simulink model "Ejercicios"  (R2023b)
settings: Solver=VariableStepAuto  StartTime=0.0  StopTime=5  MaxStep=1e-5  RelTol=1e-3
libraries: spsRMSLib x16, spsSeriesRLCBranchLib x12, spsVoltageMeasurementLib x9, spsCurrentMeasurementLib x6, spsPowerLib x6, spsACVoltageSourceLib x3, spsControlledVoltageSourceLib x2, spsDCVoltageSourceLib x1, spsDetailedThyristorLib x1, spsMutualInductanceLib x1, spsTHDLib x1, sps_lib x1
settings Model: Creator=Usuario_UMA  LastModifiedBy=Usuario_UMA

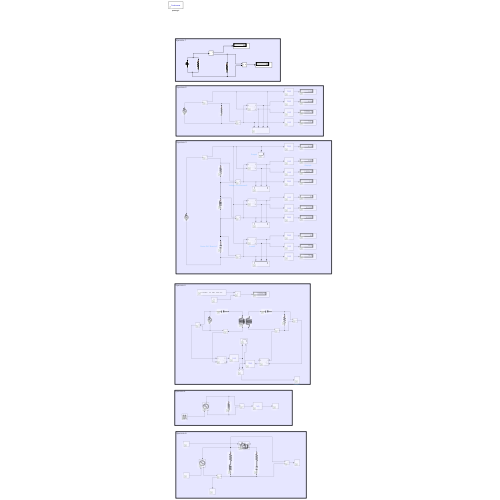
[thumbnail: Simulink's stored preview of the top-level diagram]
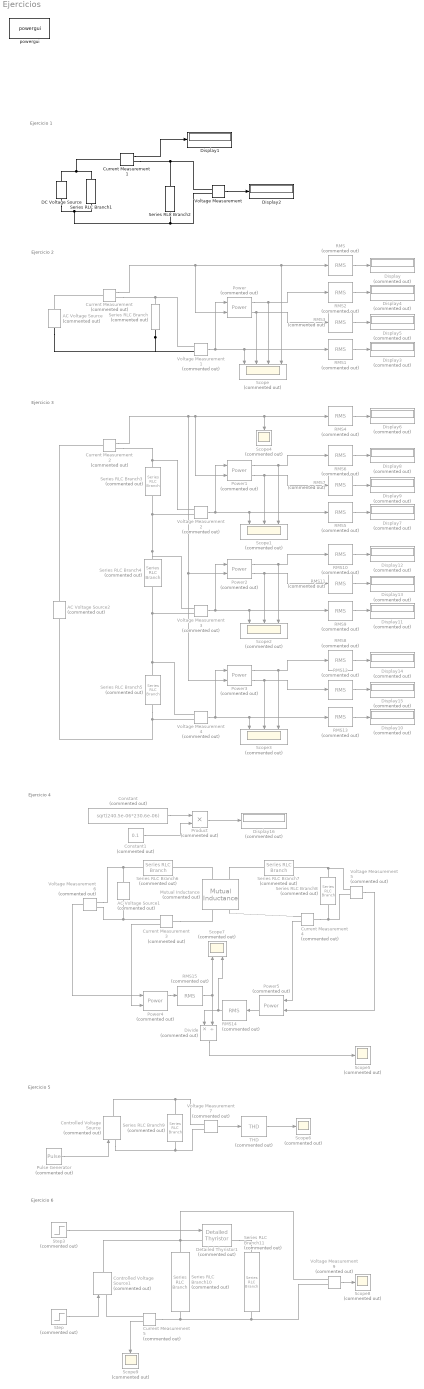
== system Ejercicios ==
  note: Ejercicio 6
  note: Ejercicio 5
  note: Ejercicio 4
  note: Ejercicio 2
  note: Ejercicio 1
  note: Ejercicio 3
  AC Voltage Source : spsACVoltageSourceLib/AC Voltage Source  Commented=on  Amplitude=10  Phase=0  Frequency=50  SampleTime=0  Measurements=None  BusType=swing  Pref=10e3  Qref=0  Qmin=-inf  Qmax=+inf
  AC Voltage Source1 : spsACVoltageSourceLib/AC Voltage Source  Commented=on  Amplitude=300  Phase=0  Frequency=85000  SampleTime=0  Measurements=None  BusType=swing  Pref=10e3  Qref=0  Qmin=-inf  Qmax=+inf
  AC Voltage Source2 : spsACVoltageSourceLib/AC Voltage Source  Commented=on  Amplitude=100  Phase=0  Frequency=50  SampleTime=0  Measurements=None  BusType=swing  Pref=10e3  Qref=0  Qmin=-inf  Qmax=+inf
  Constant : Constant  Commented=on  Value=sqrt(240.5e-06*230.6e-06)
  Constant1 : Constant  Commented=on  Value=0.1
  Controlled Voltage Source : spsControlledVoltageSourceLib/Controlled Voltage Source  Commented=on  Initialize=on  Source_Type=AC  Amplitude=0  Phase=0  Frequency=0  Measurements=None
  Controlled Voltage Source1 : spsControlledVoltageSourceLib/Controlled Voltage Source  Commented=on  Initialize=on  Source_Type=AC  Amplitude=0  Phase=0  Frequency=0  Measurements=None
  Current Measurement{,2..5} (5 alike) : spsCurrentMeasurementLib/Current Measurement  Commented=on  PhasorSimulation=off  OutputType=Complex  PSBequivalent=0
  Current Measurement1 : spsCurrentMeasurementLib/Current Measurement  PhasorSimulation=off  OutputType=Complex  PSBequivalent=0
  DC Voltage Source : spsDCVoltageSourceLib/DC Voltage Source  Amplitude=12  Measurements=None
  Detailed Thyristor1 : spsDetailedThyristorLib/Detailed Thyristor  Commented=on  Ron=0  Lon=1e-3  Vf=0  IL=0.1  Tq=100e-6  IC=0  Rs=500  Cs=250e-9  Measurements=on
      settings: LibrarySourceBlock=sps_lib/Power Electronics/Detailed Thyristor
  Display{,3..16} (15 alike) : Display  Commented=on
  Display1 : Display
  Display2 : Display
  Divide : Product  Commented=on  Inputs=*/
  Mutual Inductance : spsMutualInductanceLib/Mutual Inductance  Commented=on  LConnTagsString=a|b  RConnTagsString=A|B  TypeOfMutual=Two or three windings with equal mutual terms  NumberOfWindings=3  SelfImpedance1=[0 240.5e-06]  SelfImpedance2=[0 230.6e-06]  ThreeWindings=off  SelfImpedance3=[ 1.1 1.1e-03]  MutualImpedance=[0 2.355e-05]  InductanceMatrix="[1.0 0.9  0.9 ;  0.9 1.0  0.9;  0.9 0.9 1.0 ] * 1e-3"  ResistanceMatrix="[1.0 0.9  0.9 ;  0.9 1.0  0.9;  0.9 0.9 1.0 ]"  Measurements=None
      settings: LibrarySourceBlock=sps_lib/Passives/Mutual Inductance
  Power{,1..3} (4 alike) : spsPowerLib/Power  Commented=on  Freq=50  Vinit=[1, 0]  Iinit=[1, 0]  Ts=0
  Power4 : spsPowerLib/Power  Commented=on  Freq=85000  Vinit=[1, 0]  Iinit=[1, 0]  Ts=0
  Power5 : spsPowerLib/Power  Commented=on  Freq=85000  Vinit=[1, 0]  Iinit=[1, 0]  Ts=0
  Product : Product  Commented=on
  Pulse Generator : DiscretePulseGenerator  Commented=on  PulseType=Time based  Amplitude=10  Period=0.2  PulseWidth=40
  RMS{,1..13} (14 alike) : spsRMSLib/RMS  Commented=on  TrueRMS=on  Freq=50  RMSInit=120  Ts=0
  RMS14 : spsRMSLib/RMS  Commented=on  TrueRMS=on  Freq=85000  RMSInit=120  Ts=0
  RMS15 : spsRMSLib/RMS  Commented=on  TrueRMS=on  Freq=85000  RMSInit=120  Ts=0
  Scope : Scope  Commented=on  NumInputPorts=4
  Scope1 : Scope  Commented=on  NumInputPorts=3
  Scope2 : Scope  Commented=on  NumInputPorts=3
  Scope3 : Scope  Commented=on  NumInputPorts=3
  Scope{4..6,8..9} (5 alike) : Scope  Commented=on
  Scope7 : Scope  Commented=on  NumInputPorts=2
  Series RLC Branch : spsSeriesRLCBranchLib/Series RLC Branch  Commented=on  LConnTagsString=__new0  RConnTagsString=__new0  BranchType=R  Resistance=5  Inductance=1e-3  SetiL0=off  InitialCurrent=0  Capacitance=1e-6  Setx0=off  InitialVoltage=0  Measurements=None
  Series RLC Branch1 : spsSeriesRLCBranchLib/Series RLC Branch  LConnTagsString=__new0  RConnTagsString=__new0  BranchType=R  Resistance=0.5  Inductance=1e-3  SetiL0=off  InitialCurrent=0  Capacitance=1e-6  Setx0=off  InitialVoltage=0  Measurements=None
  Series RLC Branch10 : spsSeriesRLCBranchLib/Series RLC Branch  Commented=on  LConnTagsString=__new0  RConnTagsString=__new0  BranchType=RL  Resistance=0.2  Inductance=1.3e-3  SetiL0=off  InitialCurrent=0  Capacitance=32.2e-6  Setx0=off  InitialVoltage=0  Measurements=None
  Series RLC Branch11 : spsSeriesRLCBranchLib/Series RLC Branch  Commented=on  LConnTagsString=__new0  RConnTagsString=__new0  BranchType=RC  Resistance=5  Inductance=150e-6  SetiL0=off  InitialCurrent=0  Capacitance=0.5e-3  Setx0=off  InitialVoltage=0  Measurements=None
  Series RLC Branch2 : spsSeriesRLCBranchLib/Series RLC Branch  LConnTagsString=__new0  RConnTagsString=__new0  BranchType=R  Resistance=15  Inductance=1e-3  SetiL0=off  InitialCurrent=0  Capacitance=1e-6  Setx0=off  InitialVoltage=0  Measurements=None
  Series RLC Branch3 : spsSeriesRLCBranchLib/Series RLC Branch  Commented=on  LConnTagsString=__new0  RConnTagsString=__new0  BranchType=R  Resistance=10  Inductance=150e-6  SetiL0=off  InitialCurrent=0  Capacitance=32.2e-6  Setx0=off  InitialVoltage=0  Measurements=None
  Series RLC Branch4 : spsSeriesRLCBranchLib/Series RLC Branch  Commented=on  LConnTagsString=__new0  RConnTagsString=__new0  BranchType=L  Resistance=10  Inductance=150e-6  SetiL0=off  InitialCurrent=0  Capacitance=32.2e-6  Setx0=off  InitialVoltage=0  Measurements=None
  Series RLC Branch5 : spsSeriesRLCBranchLib/Series RLC Branch  Commented=on  LConnTagsString=__new0  RConnTagsString=__new0  BranchType=C  Resistance=10  Inductance=150e-6  SetiL0=off  InitialCurrent=0  Capacitance=32.2e-6  Setx0=off  InitialVoltage=0  Measurements=None
  Series RLC Branch6 : spsSeriesRLCBranchLib/Series RLC Branch  Commented=on  LConnTagsString=__new0  RConnTagsString=__new0  BranchType=C  Resistance=10  Inductance=150e-6  SetiL0=off  InitialCurrent=0  Capacitance=17.05e-9  Setx0=off  InitialVoltage=0  Measurements=None
  Series RLC Branch7 : spsSeriesRLCBranchLib/Series RLC Branch  Commented=on  LConnTagsString=__new0  RConnTagsString=__new0  BranchType=C  Resistance=10  Inductance=150e-6  SetiL0=off  InitialCurrent=0  Capacitance=15.88e-6  Setx0=off  InitialVoltage=0  Measurements=None
  Series RLC Branch8 : spsSeriesRLCBranchLib/Series RLC Branch  Commented=on  LConnTagsString=__new0  RConnTagsString=__new0  BranchType=R  Resistance=10  Inductance=150e-6  SetiL0=off  InitialCurrent=0  Capacitance=32.2e-6  Setx0=off  InitialVoltage=0  Measurements=None
  Series RLC Branch9 : spsSeriesRLCBranchLib/Series RLC Branch  Commented=on  LConnTagsString=__new0  RConnTagsString=__new0  BranchType=R  Resistance=1  Inductance=150e-6  SetiL0=off  InitialCurrent=0  Capacitance=32.2e-6  Setx0=off  InitialVoltage=0  Measurements=None
  Step : Step  Commented=on  Time=0.2  After=10  SampleTime=0
  Step3 : Step  Commented=on  Time=3  After=10  SampleTime=0
  THD : spsTHDLib/THD  Commented=on  Freq=5  Ts=0
  Voltage Measurement : spsVoltageMeasurementLib/Voltage Measurement  PhasorSimulation=off  OutputType=Complex  PSBequivalent=0
  Voltage Measurement{1..7,9} (8 alike) : spsVoltageMeasurementLib/Voltage Measurement  Commented=on  PhasorSimulation=off  OutputType=Complex  PSBequivalent=0
  powergui : sps_lib/powergui  Priority=1  SimulationMode=Continuous  SampleTime=50e-6  frequency=60  Iterations=50  frequencyindice=0  Pbase=100e6  ErrMax=1e-4  UnitsV=kV  UnitsW=MW  buscounter=0  FunctionMessages=off  echomessages=off  EnableUseOfTLC=off  CurrentSourceSwitches=off  DisableSnubberDevices=off  DisableRonSwitches=off  DisableVfSwitches=off  DisplayEquations=off  AutomaticDiscreteSolvers=off  SolverType=Tustin/Backward Euler (TBE)  Interpol=off  ExternalGateDelay=off  methode=off  Ts=100  x0status=blocks  SPID=on  SwTol=0  HookPort=off  NonlinearTolerance=1e-4  nMaxIteration=100  ContinueOnMaxIteration=off  RestoreLinks=warning  ResistiveCurrentMeasurement=off  Frange=[0:2:500]  Ylog=off  Xlog=on  ShowGrid=off  save=off  variable=ZData  structure=0  ZoomFFT=off  StartTime=0.0  cycles=1  DisplayStyle=1  fundamental=60  FreqAxis=off  MaxFrequency=1000  frequencyindicesteady=1  RmsSteady=1  display=off
  wires:
  RMS/1 -> Display/1
  Current Measurement1/1 -> Display1/1
  Voltage Measurement/1 -> Display2/1
  Current Measurement/1 -> Power/2, RMS/1, Scope/4
  RMS1/1 -> Display3/1
  Voltage Measurement1/1 -> Power/1, RMS1/1, Scope/1
  RMS2/1 -> Display4/1
  RMS3/1 -> Display5/1
  Power/2 -> RMS3/1, Scope/2
  Power/1 -> RMS2/1, Scope/3
  Power1/2 -> RMS7/1, Scope1/2
  Power1/1 -> RMS6/1, Scope1/3
  RMS6/1 -> Display8/1
  Voltage Measurement2/1 -> Power1/1, RMS5/1, Scope1/1
  RMS4/1 -> Display6/1
  RMS7/1 -> Display9/1
  RMS5/1 -> Display7/1
  Current Measurement2/1 -> Power3/2, Power2/2, Power1/2, Scope4/1, RMS4/1
  RMS9/1 -> Display11/1
  RMS11/1 -> Display13/1
  Power2/1 -> RMS10/1, Scope2/3
  Voltage Measurement3/1 -> Power2/1, RMS9/1, Scope2/1
  Power2/2 -> RMS11/1, Scope2/2
  RMS10/1 -> Display12/1
  RMS8/1 -> Display14/1
  Voltage Measurement4/1 -> Power3/1, RMS13/1, Scope3/1
  Power3/2 -> RMS12/1, Scope3/2
  RMS12/1 -> Display15/1
  RMS13/1 -> Display10/1
  Power3/1 -> RMS8/1, Scope3/3
  Constant/1 -> Product/1
  Constant1/1 -> Product/2
  Product/1 -> Display16/1
  Power4/1 -> RMS15/1
  Power5/1 -> RMS14/1
  Divide/1 -> Scope5/1
  RMS14/1 -> Scope7/2, Divide/1
  Current Measurement4/1 -> Power5/2
  Voltage Measurement5/1 -> Power5/1
  RMS15/1 -> Scope7/1, Divide/2
  Voltage Measurement6/1 -> Power4/1
  Current Measurement3/1 -> Power4/2
  Pulse Generator/1 -> Controlled Voltage Source/1
  Voltage Measurement7/1 -> THD/1
  THD/1 -> Scope6/1
  Step/1 -> Controlled Voltage Source1/1
  Step3/1 -> Detailed Thyristor1/1
  Voltage Measurement9/1 -> Scope8/1
  Current Measurement5/1 -> Scope9/1
  connections:
  Voltage Measurement1/LConn1 -- Current Measurement/RConn1 -- Series RLC Branch/LConn1
  Series RLC Branch/RConn1 -- AC Voltage Source/LConn1 -- Voltage Measurement1/LConn2
  DC Voltage Source/RConn1 -- Current Measurement1/LConn1 -- Series RLC Branch1/LConn1
  DC Voltage Source/LConn1 -- Series RLC Branch1/RConn1 -- Voltage Measurement/LConn2 -- Series RLC Branch2/RConn1
  Current Measurement1/RConn1 -- Voltage Measurement/LConn1 -- Series RLC Branch2/LConn1
  Current Measurement/LConn1 -- AC Voltage Source/RConn1
  Series RLC Branch5/RConn1 -- Voltage Measurement4/LConn2 -- AC Voltage Source2/LConn1
  Current Measurement2/RConn1 -- Series RLC Branch3/LConn1 -- Voltage Measurement2/LConn1
  Current Measurement2/LConn1 -- AC Voltage Source2/RConn1
  Series RLC Branch4/LConn1 -- Series RLC Branch3/RConn1 -- Voltage Measurement2/LConn2 -- Voltage Measurement3/LConn1
  Series RLC Branch5/LConn1 -- Voltage Measurement4/LConn1 -- Series RLC Branch4/RConn1 -- Voltage Measurement3/LConn2
  AC Voltage Source1/RConn1 -- Voltage Measurement6/LConn1 -- Series RLC Branch6/LConn1
  Mutual Inductance/LConn1 -- Series RLC Branch6/RConn1
  Series RLC Branch8/LConn1 -- Voltage Measurement5/LConn1 -- Series RLC Branch7/RConn1
  Series RLC Branch7/LConn1 -- Mutual Inductance/LConn2
  Current Measurement3/LConn1 -- Mutual Inductance/RConn1
  Current Measurement3/RConn1 -- Voltage Measurement6/LConn2 -- AC Voltage Source1/LConn1
  Current Measurement4/RConn1 -- Mutual Inductance/RConn2
  Voltage Measurement5/LConn2 -- Current Measurement4/LConn1 -- Series RLC Branch8/RConn1
  Series RLC Branch9/LConn1 -- Controlled Voltage Source/RConn1 -- Voltage Measurement7/LConn1
  Controlled Voltage Source/LConn1 -- Series RLC Branch9/RConn1 -- Voltage Measurement7/LConn2
  Series RLC Branch10/LConn1 -- Detailed Thyristor1/LConn1 -- Voltage Measurement9/LConn1 -- Controlled Voltage Source1/RConn1
  Series RLC Branch11/RConn1 -- Voltage Measurement9/LConn2 -- Current Measurement5/LConn1 -- Series RLC Branch10/RConn1
  Detailed Thyristor1/RConn1 -- Series RLC Branch11/LConn1
  Current Measurement5/RConn1 -- Controlled Voltage Source1/LConn1
